simulink model "OBS_s_inv_int"  (R2023b)
settings: Solver=VariableStepAuto  StartTime=0.0  StopTime=20  RelTol=1e-14  AbsTol=1e-20
values from neighbouring files (symbols this model uses):
  A = [0 1; 9.81 -0.1]    [WP3.m]
  B = [0; 1]    [WP3.m]
  C = [1 0]    [WP3.m]
  K = [92.0469   14.4179]    [WP3.m]
  L = [l1; l2]    [WP3.m]
undefined symbols (not defined in the file or in its folder): Disturbo
settings Model: Creator=giova  LastModifiedBy=miche

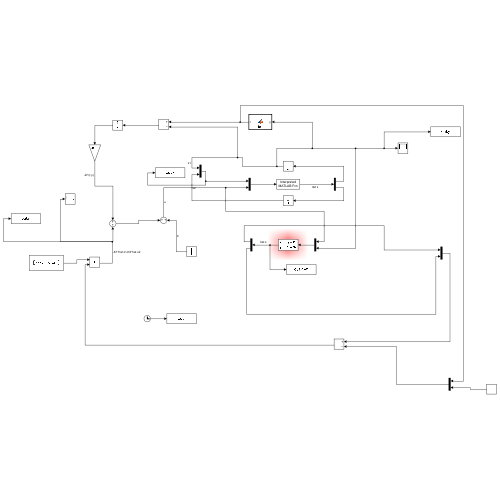
[thumbnail: Simulink's stored preview of the top-level diagram]
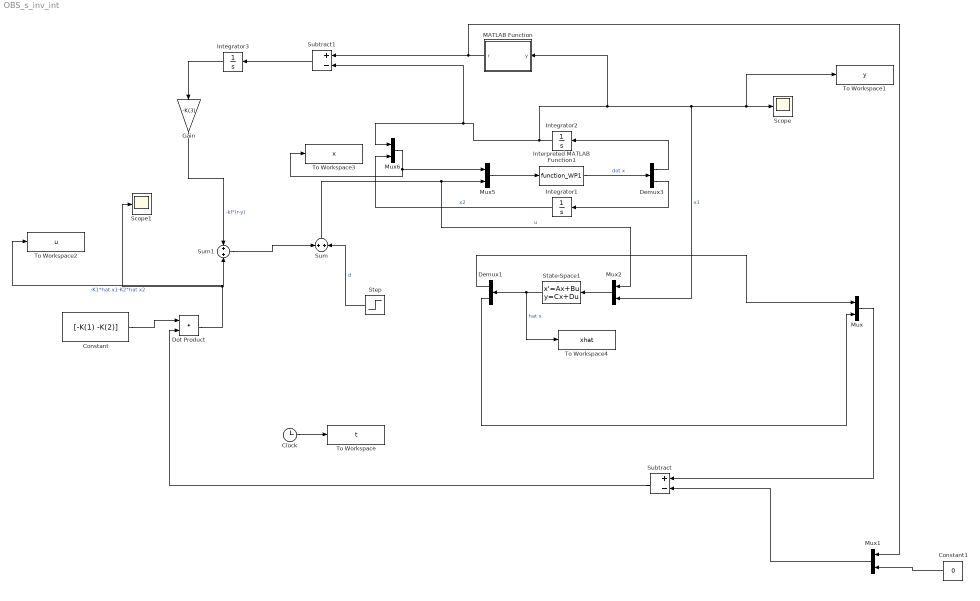
== system OBS_s_inv_int ==
  Clock : Clock
  Constant : Constant  Value=[-K(1) -K(2)]
  Constant1 : Constant  Value=0
  Demux1 : Demux  Outputs=2
  Demux3 : Demux  Outputs=2
  Dot Product : DotProduct  OutDataTypeStr=Inherit: Inherit via internal rule
  Gain : Gain  Gain=-K(3)
  Integrator1 : Integrator
  Integrator2 : Integrator
  Integrator3 : Integrator
  Interpreted MATLAB Function1 : MATLABFcn  MATLABFcn=function_WP1  OutputDimensions=2
  MATLAB Function : MATLAB Function  TreatAsAtomicUnit=on
  Mux{,1..2,5..6} (5 alike) : Mux  Inputs=2
  Scope : Scope
  Scope1 : Scope
  State-Space1 : StateSpace  A=A-L*C  B=[B L]  C=eye(2)  D=[0 0; 0 0]  InitialCondition=[0 0]
  Step : Step  Time=5  After=Disturbo  SampleTime=0
  Subtract : Sum  Inputs=+-
  Subtract1 : Sum  Inputs=+-
  Sum : Sum  Inputs=+|+
  Sum1 : Sum  Inputs=+|+
  To Workspace : ToWorkspace  VariableName=t  SampleTime=-1
  To Workspace1 : ToWorkspace  VariableName=y  SampleTime=-1
  To Workspace2 : ToWorkspace  VariableName=u  SampleTime=-1
  To Workspace3 : ToWorkspace  VariableName=x  SampleTime=-1
  To Workspace4 : ToWorkspace  VariableName=xhat  SampleTime=-1
  wires:
  Mux2/1 -> State-Space1/1
  Interpreted MATLAB Function1/1 -> Demux3/1  "dot x"
  Integrator1/1 -> Mux6/2  "x2"
  Subtract/1 -> Dot Product/2
  Demux1/2 -> Mux/2
  Mux/1 -> Subtract/1
  Dot Product/1 -> Sum1/2, To Workspace2/1, Scope1/1  "-K1*hat x1-K2*hat x2"
  Constant/1 -> Dot Product/1
  State-Space1/1 -> To Workspace4/1, Demux1/1  "hat x"
  Demux1/1 -> Mux/1
  Clock/1 -> To Workspace/1
  Integrator2/1 -> MATLAB Function/1(y), Mux2/2, To Workspace1/1, Scope/1, Subtract1/2, Mux6/1  "x1"
  Mux6/1 -> Mux5/1, To Workspace3/1
  Mux5/1 -> Interpreted MATLAB Function1/1
  Demux3/2 -> Integrator1/1
  Demux3/1 -> Integrator2/1
  Step/1 -> Sum/2  "d"
  Sum/1 -> Mux2/1, Mux5/2  "u"
  Integrator3/1 -> Gain/1
  Subtract1/1 -> Integrator3/1
  MATLAB Function/1(r) -> Subtract1/1, Mux1/1
  Gain/1 -> Sum1/1  "-kI*(r-y)"
  Sum1/1 -> Sum/1
  Mux1/1 -> Subtract/2
  Constant1/1 -> Mux1/2

== matlab function OBS_s_inv_int/MATLAB Function ==
  data: y input; r output
function r = fcn(y)
    if(y==0)
        r=pi;
    else
        r=fix(y/(2*pi))*2*pi + pi*sign(y);
    end
end
